simulink model "gm_parallel_phase_voltages_per_switching_state_6_vnl"  (R2022a)
settings: Solver=FixedStepDiscrete  StartTime=0.0  StopTime=10.0  RelTol=1e-3
undefined symbols (not defined in the file or in its folder): f_c, Rt, u_dc
libraries: hdlmdlgenlib x82, simulink x6, hdlsllib x2
(part 1 of 7)
settings Model: Creator=Andre Merx  LastModifiedBy=Andre Merx
settings SolverCC: AlgebraicLoopSolver=TrustRegion
settings DataIOCC: LimitDataPoints=on  SaveOutput=off  SaveTime=off
settings OptimizationCC: BlockReduction=off  ConditionallyExecuteInputs=off  DefaultParameterBehavior=Inlined  LifeSpan=inf
settings DebuggingCC: AlgebraicLoopMsg=error  InheritedTsInSrcMsg=none  SingleTaskRateTransMsg=error  UnconnectedInputMsg=warning  UnconnectedOutputMsg=warning  UnconnectedLineMsg=warning  AllowSymbolicDim=off  StrictBusMsg=ErrorOnBusTreatedAsVector  SFUnexpectedBacktrackingDiag=warning  SFNoUnconditionalDefaultTransitionDiag=warning  SFExecutionAtInitializationDiag=none  SFMachineParentedDataDiag=warning  ArithmeticOperatorsInVariantConditions=warning
settings HardwareCC: ProdBitPerPointer=32  ProdBitPerSizeT=32  ProdBitPerPtrDiffT=32  ProdLargestAtomicFloat=None  ProdIntDivRoundTo=Undefined  ProdEndianess=Unspecified  ProdWordSize=32  ProdHWDeviceType=ASIC/FPGA->ASIC/FPGA  ProdEqTarget=off
settings SFSimCC: SimUseLocalCustomCode=off  CustomCodeUndefinedFunction=UseInterfaceOnly
settings RTWCC: RTWUseLocalCustomCode=off
settings CodeAppCC: StateflowObjectComments=on
settings GRTTargetCC: TargetLangStandard=C89/C90 (ANSI)
settings ConfigComp: CovScope=ReferencedModels  CovMetricSettings=dw  CovSaveCumulativeToWorkspaceVar=on  CovSaveSingleToWorkspaceVar=on  CovExternalEMLEnable=off  CovSFcnEnable=off

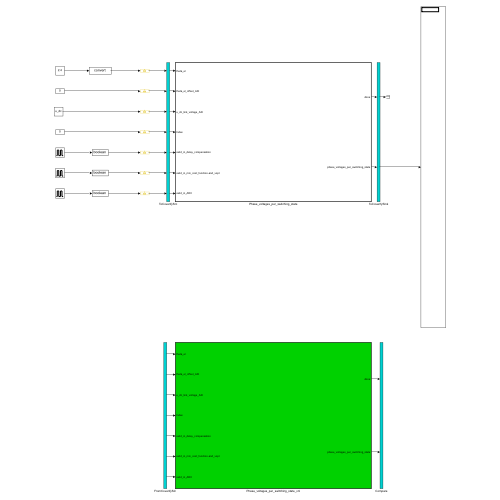
[thumbnail: Simulink's stored preview of the top-level diagram]
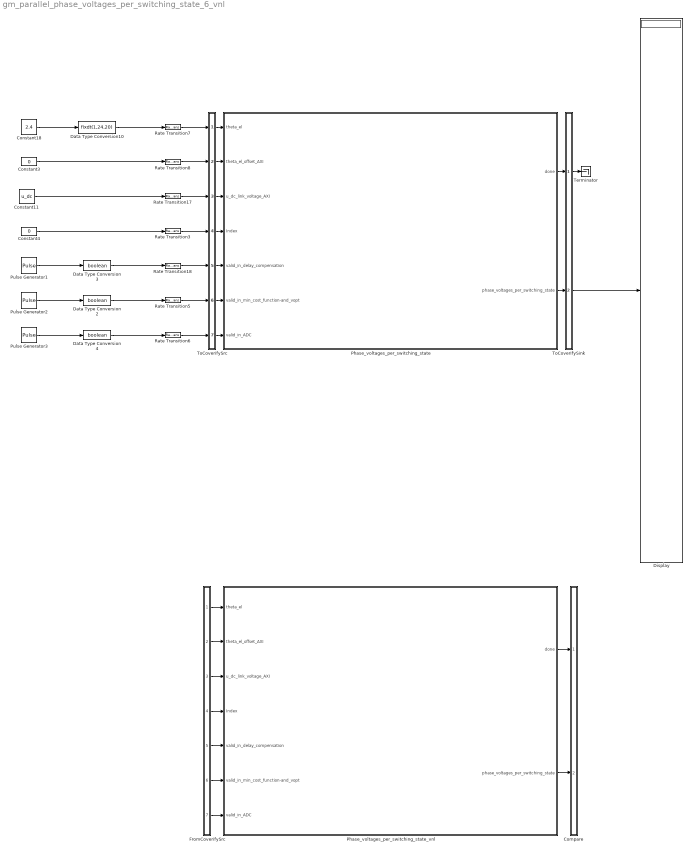
== system gm_parallel_phase_voltages_per_switching_state_6_vnl ==
  Compare : Subsystem
      mask Display: disp('')
  Constant11 : Constant  Value=u_dc  OutDataTypeStr=single  SampleTime=-1
  Constant18 : Constant  Value=2.4
  Constant3 : Constant  Value=0  OutDataTypeStr=single  SampleTime=-1
  Constant4 : Constant  Value=0  OutDataTypeStr=int32  SampleTime=-1
  Data Type Conversion10 : DataTypeConversion  OutDataTypeStr=fixdt(1,24,20)  SaturateOnIntegerOverflow=off  RndMeth=Floor
  Data Type Conversion2 : DataTypeConversion  OutDataTypeStr=boolean  SaturateOnIntegerOverflow=off  RndMeth=Floor
  Data Type Conversion3 : DataTypeConversion  OutDataTypeStr=boolean  SaturateOnIntegerOverflow=off  RndMeth=Floor
  Data Type Conversion4 : DataTypeConversion  OutDataTypeStr=boolean  SaturateOnIntegerOverflow=off  RndMeth=Floor
  Display : Display
  FromCoverifySrc : Subsystem
      mask Display: disp('')
  Phase_voltages_per_switching_state : Subsystem  TreatAsAtomicUnit=on
  Phase_voltages_per_switching_state_vnl : Subsystem  TreatAsAtomicUnit=on
  Pulse Generator1 : DiscretePulseGenerator  PulseType=Time based  Period=1/f_c
  Pulse Generator2 : DiscretePulseGenerator  PulseType=Time based  Period=1/f_c
  Pulse Generator3 : DiscretePulseGenerator  PulseType=Time based  Period=1/f_c
  Rate Transition{3,5..8,17..18} (7 alike) : RateTransition  OutPortSampleTime=Rt
  Terminator : Terminator
  ToCoverifySink : Subsystem
      mask Display: disp('')
  ToCoverifySrc : Subsystem
      mask Display: disp('')
  wires:
  Data Type Conversion2/1 -> Rate Transition5/1
  Data Type Conversion3/1 -> Rate Transition18/1
  Data Type Conversion4/1 -> Rate Transition6/1
  Pulse Generator3/1 -> Data Type Conversion4/1
  Pulse Generator2/1 -> Data Type Conversion2/1
  Constant18/1 -> Data Type Conversion10/1
  Pulse Generator1/1 -> Data Type Conversion3/1
  Constant4/1 -> Rate Transition3/1
  Constant3/1 -> Rate Transition8/1
  Constant11/1 -> Rate Transition17/1
  Data Type Conversion10/1 -> Rate Transition7/1
  ToCoverifySrc/1(out1) -> Phase_voltages_per_switching_state/1(theta_el)
  ToCoverifySrc/2(out2) -> Phase_voltages_per_switching_state/2(theta_el_offset_AXI)
  ToCoverifySrc/3(out3) -> Phase_voltages_per_switching_state/3(u_dc_link_voltage_AXI)
  ToCoverifySrc/4(out4) -> Phase_voltages_per_switching_state/4(Index)
  ToCoverifySrc/5(out5) -> Phase_voltages_per_switching_state/5(valid_in_delay_compensation)
  ToCoverifySrc/6(out6) -> Phase_voltages_per_switching_state/6(valid_in_min_cost_function-and_vopt)
  ToCoverifySrc/7(out7) -> Phase_voltages_per_switching_state/7(valid_in_ADC)
  Phase_voltages_per_switching_state/1(done) -> ToCoverifySink/1(in1)
  Phase_voltages_per_switching_state/2(phase_voltages_per_switching_state) -> ToCoverifySink/2(in2)
  Rate Transition7/1 -> ToCoverifySrc/1(in1)
  Rate Transition8/1 -> ToCoverifySrc/2(in2)
  Rate Transition17/1 -> ToCoverifySrc/3(in3)
  Rate Transition3/1 -> ToCoverifySrc/4(in4)
  Rate Transition18/1 -> ToCoverifySrc/5(in5)
  Rate Transition5/1 -> ToCoverifySrc/6(in6)
  Rate Transition6/1 -> ToCoverifySrc/7(in7)
  ToCoverifySink/1(out1) -> Terminator/1
  ToCoverifySink/2(out2) -> Display/1
  FromCoverifySrc/1(out1) -> Phase_voltages_per_switching_state_vnl/1(theta_el)
  FromCoverifySrc/2(out2) -> Phase_voltages_per_switching_state_vnl/2(theta_el_offset_AXI)
  FromCoverifySrc/3(out3) -> Phase_voltages_per_switching_state_vnl/3(u_dc_link_voltage_AXI)
  FromCoverifySrc/4(out4) -> Phase_voltages_per_switching_state_vnl/4(Index)
  FromCoverifySrc/5(out5) -> Phase_voltages_per_switching_state_vnl/5(valid_in_delay_compensation)
  FromCoverifySrc/6(out6) -> Phase_voltages_per_switching_state_vnl/6(valid_in_min_cost_function-and_vopt)
  FromCoverifySrc/7(out7) -> Phase_voltages_per_switching_state_vnl/7(valid_in_ADC)
  Phase_voltages_per_switching_state_vnl/1(done) -> Compare/1(in1)
  Phase_voltages_per_switching_state_vnl/2(phase_voltages_per_switching_state) -> Compare/2(in2)

== system gm_parallel_phase_voltages_per_switching_state_6_vnl/Compare ==
  in1 : Inport
  in2 : Inport  Port=2
  Assert_done : Subsystem
  Assert_phase_voltages_per_switching_state : Subsystem
  CleanupScopes : Subsystem
      settings: OpenFcn=|
      | blkName = gcb; %self block
      | idx = regexp(blkName, '/CleanupScopes$', 'once');
      | blkParent = blkName(1:idx-1);
      | blks=find_system(blkParent, 'LookUnderMasks', 'all','blocktype', 'Scope');
      | for itr = 1:length(blks)
      | 	 hScopeCfg = get_param(blks{itr},'ScopeConfiguration');
      | 	 hScopeCfg.Visible = ~ hScopeCfg.Visible;
      | end
      | drawnow;
      mask Display: fprintf(message('hdlcoder:cosim:vnl_dblclick').getString());
  Enable : Subsystem
      settings: OpenFcn=|
      | blkName = gcb;
      | idx = regexp(blkName, '/Enable$', 'once');
      | blkParent = blkName(1:idx-1);
      | blks=find_system(blkParent, 'LookUnderMasks', 'all','blocktype', 'Assertion');
      | e = get_param(blks{1}, 'Enabled');
      | if strcmp(e, 'on'), f= 'off';, else, f = 'on';, end
      | for ii=1:length(blks), set_param(blks{ii}, 'Enabled', f);, end
      | set_param(gcb, 'MaskDisplay',['fprintf(message(''hdlcoder:cosim:vnl_dblclick_assertions'',','''',upper(e),'''',').getString())']);
      mask Display: fprintf(message('hdlcoder:cosim:vnl_dblclick_assertions','OFF').getString());
  pathdelay1 : Delay  DelayLength=68
  pathdelay2 : Delay  DelayLength=68
  wires:
  in1/1 -> pathdelay1/1
  pathdelay1/1 -> Assert_done/1(cosim)
  [out1] -> Assert_done/2(dut)
  in2/1 -> pathdelay2/1
  pathdelay2/1 -> Assert_phase_voltages_per_switching_state/1(cosim)
  [out2] -> Assert_phase_voltages_per_switching_state/2(dut)

== system gm_parallel_phase_voltages_per_switching_state_6_vnl/FromCoverifySrc ==
  out1 : Outport
  out2 : Outport  Port=2
  out3 : Outport  Port=3
  out4 : Outport  Port=4
  out5 : Outport  Port=5
  out6 : Outport  Port=6
  out7 : Outport  Port=7
  wires:
  [in1] -> out1/1
  [in2] -> out2/1
  [in3] -> out3/1
  [in4] -> out4/1
  [in5] -> out5/1
  [in6] -> out6/1
  [in7] -> out7/1

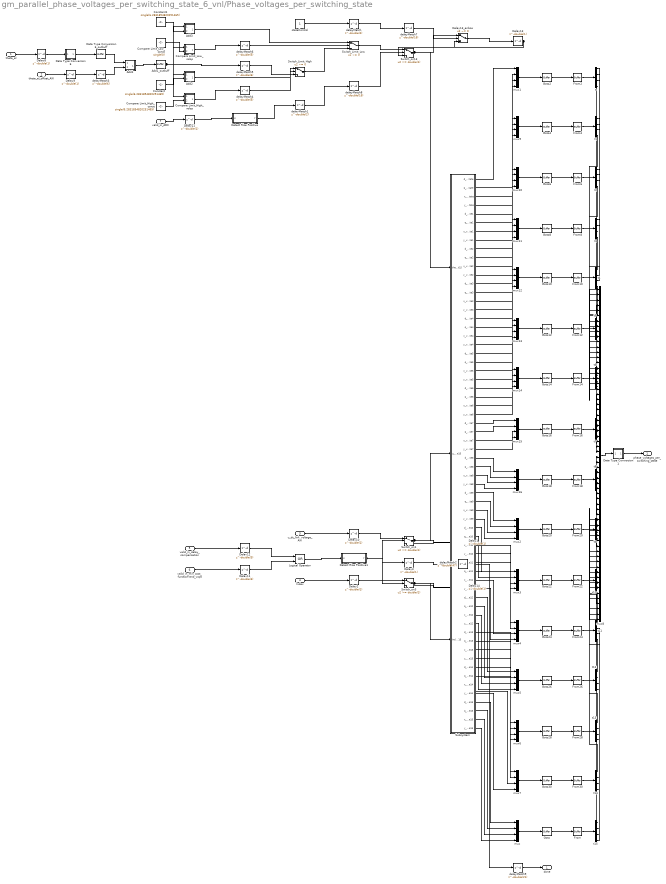
== system gm_parallel_phase_voltages_per_switching_state_6_vnl/Phase_voltages_per_switching_state ==
  theta_el : Inport  OutDataTypeStr=fixdt(1, 24, 20)  PortDimensions=1  SampleTime=1e-08
  theta_el_offset_AXI : Inport  Port=2  OutDataTypeStr=single  PortDimensions=1  SampleTime=1e-08
  u_dc_link_voltage_AXI : Inport  Port=3  OutDataTypeStr=single  PortDimensions=1  SampleTime=1e-08
  Index : Inport  Port=4  OutDataTypeStr=int32  PortDimensions=1  SampleTime=1e-08
  valid_in_delay_compensation : Inport  Port=5  OutDataTypeStr=boolean  PortDimensions=1  SampleTime=1e-08
  valid_in_min_cost_function-and_vopt : Inport  Port=6  OutDataTypeStr=boolean  PortDimensions=1  SampleTime=1e-08
  valid_in_ADC : Inport  Port=7  OutDataTypeStr=boolean  PortDimensions=1  SampleTime=1e-08
  Add1 : Subsystem
      mask Display: disp('NFP\nadd');
  Add1_outbuff : hdlmdlgenlib/Buffer
      settings: SourceProductBaseCode=SL
  Add2 : Subsystem
      mask Display: disp('NFP\nadd');
  Add3 : Subsystem
      mask Display: disp('NFP\nadd');
  Compare Limit_High_const : Constant  Value=single(6.2831854820251465)  OutDataTypeStr=single  SampleTime=1e-08
  Compare Limit_High_relop : Subsystem
      mask Display: disp('NFP\nrelop');
  Compare Limit_Low_const : Constant  Value=single(0)  OutDataTypeStr=single  SampleTime=1e-08
  Compare Limit_Low_relop : Subsystem
      mask Display: disp('NFP\nrelop');
  Constant : Constant  Value=single(6.2831854820251465)  OutDataTypeStr=single  SampleTime=1e-08
  Constant1 : Constant  Value=single(6.2831854820251465)  OutDataTypeStr=single  SampleTime=1e-08
  Data Type Conversion1 : Subsystem
      mask Display: disp('NFP\nconv');
  Data Type Conversion6 : Subsystem
      mask Display: disp('NFP\nconv');
  Data Type Conversion6_outbuff : hdlmdlgenlib/Buffer
      settings: SourceProductBaseCode=SL
  Delay{1..3,8..10,13..14,21} (9 alike) : Delay  DelayLength=double(1)  InitialCondition=0  SampleTime=1e-08
  Delay11 : Delay  DelayLength=double(3)  InitialCondition=0  SampleTime=1e-08
  Delay12 : Delay  DelayLength=double(3)  InitialCondition=0  SampleTime=1e-08
  Delay13_enbsw : Switch  Criteria=u2 ~= 0  Threshold=double(0)  OutDataTypeStr=single  SampleTime=1e-08  SaturateOnIntegerOverflow=off  InputSameDT=off
  Detect Rise Positive : Subsystem  mask(Detect Rise Positive){vinit=double(0), InputProcessing=Elements as channels (sample based), OutDataTypeStr=boolean}
      mask prompts: vinit "Simulink:masks:InitialCondition_MP"; InputProcessing "Simulink:masks:InputProcessing_MP"; OutDataTypeStr "Simulink:masks:OutputDataType_MP"
      mask help: Simulink:masks:DetectRisePositive_MD
      mask init:
      | InputProcessing = 'Elements as channels (sample based)';
      | OutDataTypeStr = 'boolean';
      | vinit = double(0);
      mask TypeOptions InputProcessing: Simulink:masks:ColumnsAsChannelsFrameBased | Simulink:masks:ElementsAsChannelsSampleBased
      mask TypeOptions OutDataTypeStr: Simulink:masks:uint8 | Simulink:masks:boolean
      mask Display: fprintf('U > 0\n&  NOT\nU/z > 0')
  Detect Rise Positive1 : Subsystem  mask(Detect Rise Positive){vinit=double(0), InputProcessing=Elements as channels (sample based), OutDataTypeStr=boolean}
      mask prompts: vinit "Simulink:masks:InitialCondition_MP"; InputProcessing "Simulink:masks:InputProcessing_MP"; OutDataTypeStr "Simulink:masks:OutputDataType_MP"
      mask help: Simulink:masks:DetectRisePositive_MD
      mask init:
      | InputProcessing = 'Elements as channels (sample based)';
      | OutDataTypeStr = 'boolean';
      | vinit = double(0);
      mask TypeOptions InputProcessing: Simulink:masks:ColumnsAsChannelsFrameBased | Simulink:masks:ElementsAsChannelsSampleBased
      mask TypeOptions OutDataTypeStr: Simulink:masks:uint8 | Simulink:masks:boolean
      mask Display: fprintf('U > 0\n&  NOT\nU/z > 0')
  From{,2,4,6,8,10,12,14,16,18,20,22,24,26,28,30} (16 alike) : hdlmdlgenlib/Buffer
      settings: SourceProductBaseCode=SL
  Goto{,2,4,6,8,10,12,14,16,18,20,22,24,26,28,30} (16 alike) : hdlmdlgenlib/Buffer
      settings: SourceProductBaseCode=SL
  Logical Operator : Logic  Operator=OR  AllPortsSameDT=off  OutDataTypeStr=boolean  SampleTime=1e-08
  Subsystem : Subsystem
  Switch_Limit_High : Switch  Criteria=u2 ~= 0  Threshold=double(0)  OutDataTypeStr=single  SampleTime=1e-08  SaturateOnIntegerOverflow=off  InputSameDT=off
  Switch_Limit_Low : Switch  Criteria=u2 ~= 0  Threshold=double(0)  OutDataTypeStr=single  SampleTime=1e-08  SaturateOnIntegerOverflow=off  InputSameDT=off
  Switch_on1 : Switch  Threshold=double(1)  OutDataTypeStr=single  RndMeth=Simplest  SampleTime=1e-08  SaturateOnIntegerOverflow=off  InputSameDT=off
  Switch_on13 : Switch  Threshold=double(1)  OutDataTypeStr=single  RndMeth=Simplest  SampleTime=1e-08  SaturateOnIntegerOverflow=off  InputSameDT=off
  Switch_on3 : Switch  Threshold=double(1)  OutDataTypeStr=int32  RndMeth=Simplest  SampleTime=1e-08  SaturateOnIntegerOverflow=off  InputSameDT=off
  delayMatch : Delay  DelayLength=double(2)  InitialCondition=0  SampleTime=1e-08
  delayMatch1 : Delay  DelayLength=double(2)  InitialCondition=0  SampleTime=1e-08
  delayMatch2 : Delay  DelayLength=double(47)  InitialCondition=0  SampleTime=1e-08
  delayMatch3 : Delay  DelayLength=double(6)  InitialCondition=0  SampleTime=1e-08
  delayMatch4 : Delay  DelayLength=double(5)  InitialCondition=0  SampleTime=1e-08
  delayMatch5 : Delay  DelayLength=double(6)  InitialCondition=0  SampleTime=1e-08
  delayMatch6 : Delay  DelayLength=double(5)  InitialCondition=0  SampleTime=1e-08
  delayMatch7 : Delay  DelayLength=double(16)  InitialCondition=0  SampleTime=1e-08
  delayMatch8 : Delay  DelayLength=double(16)  InitialCondition=0  SampleTime=1e-08
  delayMatch9 : Delay  DelayLength=double(21)  InitialCondition=0  SampleTime=1e-08
  mux{,1..7,9..16} (16 alike) : Mux
  mux8 : Mux  Inputs=64
  stateControl : Constant  OutDataTypeStr=boolean  SampleTime=1e-08
  t{,1..15} (16 alike) : Demux
  done : Outport  SampleTime=1e-08
  phase_voltages_per_switching_state : Outport  Port=2  SampleTime=1e-08
  wires:
  Delay14/1 -> Switch_on3/3
  Delay1/1 -> Switch_on1/3
  Delay13/1 -> Delay13_enbsw/3, Switch_on13/3
  Delay13_enbsw/1 -> Delay13/1
  Switch_on13/1 -> Delay13_enbsw/1, Subsystem/1(theta_el_with_offset15)
  delayMatch2/1 -> delayMatch9/1
  delayMatch1/1 -> delayMatch8/1
  delayMatch/1 -> delayMatch7/1
  Delay9/1 -> delayMatch3/1
  Data Type Conversion6/1(Out1) -> Data Type Conversion6_outbuff/1
  Data Type Conversion1/1(Out1) -> phase_voltages_per_switching_state/1
  Compare Limit_Low_relop/1(Out1) -> delayMatch6/1
  Compare Limit_High_relop/1(Out1) -> delayMatch4/1
  Add3/1(Out1) -> Switch_Limit_Low/1
  Add2/1(Out1) -> Switch_Limit_High/1
  Add1/1(Out1) -> Add1_outbuff/1
  Delay3/1 -> delayMatch2/1
  Detect Rise Positive/1(Y) -> delayMatch1/1
  stateControl/1 -> delayMatch/1
  delayMatch7/1 -> Delay13_enbsw/2
  t15/4 -> mux8/64
  t15/3 -> mux8/63
  t15/2 -> mux8/62
  t15/1 -> mux8/61
  t14/4 -> mux8/60
  t14/3 -> mux8/59
  t14/2 -> mux8/58
  t14/1 -> mux8/57
  t13/4 -> mux8/56
  t13/3 -> mux8/55
  t13/2 -> mux8/54
  t13/1 -> mux8/53
  t12/4 -> mux8/52
  t12/3 -> mux8/51
  t12/2 -> mux8/50
  t12/1 -> mux8/49
  t11/4 -> mux8/48
  t11/3 -> mux8/47
  t11/2 -> mux8/46
  t11/1 -> mux8/45
  t10/4 -> mux8/44
  t10/3 -> mux8/43
  t10/2 -> mux8/42
  t10/1 -> mux8/41
  t9/4 -> mux8/40
  t9/3 -> mux8/39
  t9/2 -> mux8/38
  t9/1 -> mux8/37
  t8/4 -> mux8/36
  t8/3 -> mux8/35
  t8/2 -> mux8/34
  t8/1 -> mux8/33
  t7/4 -> mux8/32
  t7/3 -> mux8/31
  t7/2 -> mux8/30
  t7/1 -> mux8/29
  t6/4 -> mux8/28
  t6/3 -> mux8/27
  t6/2 -> mux8/26
  t6/1 -> mux8/25
  t5/4 -> mux8/24
  t5/3 -> mux8/23
  t5/2 -> mux8/22
  t5/1 -> mux8/21
  t4/4 -> mux8/20
  t4/3 -> mux8/19
  t4/2 -> mux8/18
  t4/1 -> mux8/17
  t3/4 -> mux8/16
  t3/3 -> mux8/15
  t3/2 -> mux8/14
  t3/1 -> mux8/13
  t2/4 -> mux8/12
  t2/3 -> mux8/11
  t2/2 -> mux8/10
  t2/1 -> mux8/9
  t1/4 -> mux8/8
  t1/3 -> mux8/7
  t1/2 -> mux8/6
  t1/1 -> mux8/5
  t/4 -> mux8/4
  t/3 -> mux8/3
  t/2 -> mux8/2
  t/1 -> mux8/1
  Compare Limit_Low_const/1 -> Compare Limit_Low_relop/2(In2)
  Compare Limit_High_const/1 -> Compare Limit_High_relop/2(In2)
  delayMatch6/1 -> Switch_Limit_Low/2
  delayMatch4/1 -> Switch_Limit_High/2
  Add1_outbuff/1 -> delayMatch5/1, Add2/1(In1), Add3/1(In1), Compare Limit_High_relop/1(In1), Compare Limit_Low_relop/1(In1)
  Goto8/1 -> From8/1
  Goto6/1 -> From6/1
  Goto4/1 -> From4/1
  Goto30/1 -> From30/1
  Goto28/1 -> From28/1
  Goto26/1 -> From26/1
  Goto24/1 -> From24/1
  Goto22/1 -> From22/1
  Goto20/1 -> From20/1
  Goto2/1 -> From2/1
  Goto18/1 -> From18/1
  Goto16/1 -> From16/1
  Goto14/1 -> From14/1
  Goto12/1 -> From12/1
  Goto10/1 -> From10/1
  Goto/1 -> From/1
  Switch_on3/1 -> Delay14/1, Subsystem/3(Index 15)
  Switch_on1/1 -> Delay1/1, Subsystem/2(u_dc_link_voltage15)
  Switch_Limit_Low/1 -> Switch_on13/1
  Switch_Limit_High/1 -> Switch_Limit_Low/3
  Subsystem/64(y_voltage_per_switching_state15) -> mux/4
  Subsystem/63(x_voltage_per_switching_state15) -> mux/3
  Subsystem/62(q_voltage_per_switching_state15) -> mux/2
  Subsystem/61(d_voltage_per_switching_state15) -> mux/1
  Subsystem/60(y_voltage_per_switching_state14) -> mux7/4
  Subsystem/59(x_voltage_per_switching_state14) -> mux7/3
  Subsystem/58(q_voltage_per_switching_state14) -> mux7/2
  Subsystem/57(d_voltage_per_switching_state14) -> mux7/1
  Subsystem/56(y_voltage_per_switching_state13) -> mux6/4
  Subsystem/55(x_voltage_per_switching_state13) -> mux6/3
  Subsystem/54(q_voltage_per_switching_state13) -> mux6/2
  Subsystem/53(d_voltage_per_switching_state13) -> mux6/1
  Subsystem/52(y_voltage_per_switching_state12) -> mux5/4
  Subsystem/51(x_voltage_per_switching_state12) -> mux5/3
  Subsystem/50(q_voltage_per_switching_state12) -> mux5/2
  Subsystem/49(d_voltage_per_switching_state12) -> mux5/1
  Subsystem/48(y_voltage_per_switching_state11) -> mux4/4
  Subsystem/47(x_voltage_per_switching_state11) -> mux4/3
  Subsystem/46(q_voltage_per_switching_state11) -> mux4/2
  Subsystem/45(d_voltage_per_switching_state11) -> mux4/1
  Subsystem/44(y_voltage_per_switching_state10) -> mux3/4
  Subsystem/43(x_voltage_per_switching_state10) -> mux3/3
  Subsystem/42(q_voltage_per_switching_state10) -> mux3/2
  Subsystem/41(d_voltage_per_switching_state10) -> mux3/1
  Subsystem/40(y_voltage_per_switching_state9) -> mux2/4
  Subsystem/39(x_voltage_per_switching_state9) -> mux2/3
  Subsystem/38(q_voltage_per_switching_state9) -> mux2/2
  Subsystem/37(d_voltage_per_switching_state9) -> mux2/1
  Subsystem/36(y_voltage_per_switching_state8) -> mux16/4
  Subsystem/35(x_voltage_per_switching_state8) -> mux16/3
  Subsystem/34(q_voltage_per_switching_state8) -> mux16/2
  Subsystem/33(d_voltage_per_switching_state8) -> mux16/1
  Subsystem/32(y_voltage_per_switching_state7) -> mux15/4
  Subsystem/31(x_voltage_per_switching_state7) -> mux15/3
  Subsystem/30(q_voltage_per_switching_state7) -> mux15/2
  Subsystem/29(d_voltage_per_switching_state7) -> mux15/1
  Subsystem/28(y_voltage_per_switching_state6) -> mux14/4
  Subsystem/27(x_voltage_per_switching_state6) -> mux14/3
  Subsystem/26(q_voltage_per_switching_state6) -> mux14/2
  Subsystem/25(d_voltage_per_switching_state6) -> mux14/1
  Subsystem/24(y_voltage_per_switching_state5) -> mux13/4
  Subsystem/23(x_voltage_per_switching_state5) -> mux13/3
  Subsystem/22(q_voltage_per_switching_state5) -> mux13/2
  Subsystem/21(d_voltage_per_switching_state5) -> mux13/1
  Subsystem/20(y_voltage_per_switching_state4) -> mux12/4
  Subsystem/19(x_voltage_per_switching_state4) -> mux12/3
  Subsystem/18(q_voltage_per_switching_state4) -> mux12/2
  Subsystem/17(d_voltage_per_switching_state4) -> mux12/1
  Subsystem/16(y_voltage_per_switching_state3) -> mux11/4
  Subsystem/15(x_voltage_per_switching_state3) -> mux11/3
  Subsystem/14(q_voltage_per_switching_state3) -> mux11/2
  Subsystem/13(d_voltage_per_switching_state3) -> mux11/1
  Subsystem/12(y_voltage_per_switching_state2) -> mux10/4
  Subsystem/11(x_voltage_per_switching_state2) -> mux10/3
  Subsystem/10(q_voltage_per_switching_state2) -> mux10/2
  Subsystem/9(d_voltage_per_switching_state2) -> mux10/1
  Subsystem/8(y_voltage_per_switching_state1) -> mux9/4
  Subsystem/7(x_voltage_per_switching_state1) -> mux9/3
  Subsystem/6(q_voltage_per_switching_state1) -> mux9/2
  Subsystem/5(d_voltage_per_switching_state1) -> mux9/1
  Subsystem/4(y_voltage_per_switching_state) -> mux1/4
  Subsystem/3(x_voltage_per_switching_state) -> mux1/3
  Subsystem/2(q_voltage_per_switching_state) -> mux1/2
  Subsystem/1(d_voltage_per_switching_state) -> mux1/1
  mux16/1 -> Goto18/1
  mux15/1 -> Goto16/1
  mux14/1 -> Goto14/1
  mux13/1 -> Goto12/1
  mux12/1 -> Goto10/1
  mux11/1 -> Goto8/1
  mux10/1 -> Goto6/1
  mux9/1 -> Goto4/1
  mux8/1 -> Data Type Conversion1/1(In1)
  mux7/1 -> Goto30/1
  mux6/1 -> Goto28/1
  mux5/1 -> Goto26/1
  mux4/1 -> Goto24/1
  mux3/1 -> Goto22/1
  mux2/1 -> Goto20/1
  mux1/1 -> Goto2/1
  mux/1 -> Goto/1
  Logical Operator/1 -> Detect Rise Positive1/1(U)
  From8/1 -> t3/1
  From6/1 -> t2/1
  From4/1 -> t1/1
  From30/1 -> t14/1
  From28/1 -> t13/1
  From26/1 -> t12/1
  From24/1 -> t11/1
  From22/1 -> t10/1
  From20/1 -> t9/1
  From2/1 -> t/1
  From18/1 -> t8/1
  From16/1 -> t7/1
  From14/1 -> t6/1
  From12/1 -> t5/1
  From10/1 -> t4/1
  From/1 -> t15/1
  Detect Rise Positive1/1(Y) -> Switch_on3/2, Switch_on1/2, Delay3/1
  delayMatch8/1 -> Switch_on13/2
  delayMatch3/1 -> Add1/2(In2)
  Delay8/1 -> Data Type Conversion6/1(In1)
  delayMatch9/1 -> done/1
  Delay21/1 -> Detect Rise Positive/1(U)
  Delay2/1 -> Switch_on3/1
  Delay12/1 -> Logical Operator/1
  Delay11/1 -> Logical Operator/2
  Delay10/1 -> Switch_on1/1
  Data Type Conversion6_outbuff/1 -> Add1/1(In1)
  Constant1/1 -> Add3/2(In2)
  Constant/1 -> Add2/2(In2)
  delayMatch5/1 -> Switch_Limit_High/3
  valid_in_ADC/1 -> Delay21/1
  valid_in_min_cost_function-and_vopt/1 -> Delay11/1
  valid_in_delay_compensation/1 -> Delay12/1
  Index/1 -> Delay2/1
  u_dc_link_voltage_AXI/1 -> Delay10/1
  theta_el_offset_AXI/1 -> Delay9/1
  theta_el/1 -> Delay8/1

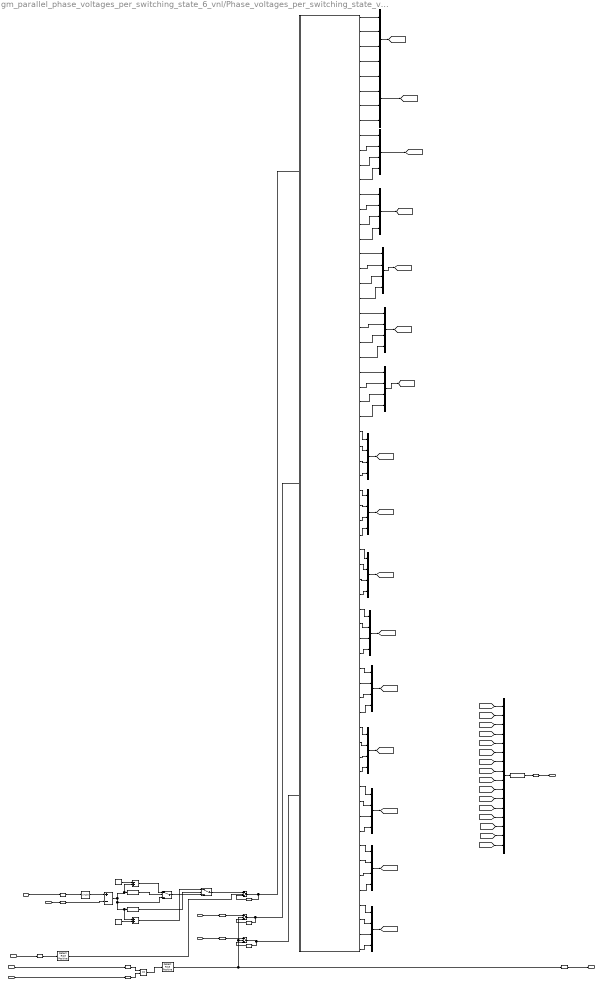
== system gm_parallel_phase_voltages_per_switching_state_6_vnl/Phase_voltages_per_switching_state_vnl ==
  theta_el : Inport
  theta_el_offset_AXI : Inport  Port=2
  u_dc_link_voltage_AXI : Inport  Port=3
  Index : Inport  Port=4
  valid_in_delay_compensation : Inport  Port=5
  valid_in_min_cost_function-and_vopt : Inport  Port=6
  valid_in_ADC : Inport  Port=7
  Add1 : Sum  Inputs=+-  OutDataTypeStr=Inherit: Same as accumulator
  Add2 : Sum  Inputs=-+  OutDataTypeStr=Inherit: Same as first input
  Add3 : Sum  OutDataTypeStr=Inherit: Same as first input
  Compare Limit_High : simulink/Logic and Bit Operations/Compare To Constant  relop=>=  const=2*pi  OutDataTypeStr=boolean
  Compare Limit_Low : simulink/Logic and Bit Operations/Compare To Constant  relop=<  const=0  OutDataTypeStr=boolean
  Constant : Constant  Value=2*pi  OutDataTypeStr=single  SampleTime=Rt
  Constant1 : Constant  Value=2*pi  OutDataTypeStr=single  SampleTime=Rt
  Data Type Conversion1 : DataTypeConversion  OutDataTypeStr=fixdt(1,24,11)  SaturateOnIntegerOverflow=off  RndMeth=Floor
  Data Type Conversion6 : DataTypeConversion  OutDataTypeStr=single  RndMeth=Nearest  SaturateOnIntegerOverflow=off
  Delay{1..4,8..10,13..14,21} (10 alike) : Delay  DelayLength=1
  Delay11 : Delay  DelayLength=3
  Delay12 : Delay  DelayLength=3
  Detect Rise Positive : hdlsllib/Logic and Bit Operations/Detect Rise Positive  vinit=0  OutDataTypeStr=boolean
      settings: SourceProductBaseCode=SL
  Detect Rise Positive1 : hdlsllib/Logic and Bit Operations/Detect Rise Positive  vinit=0  OutDataTypeStr=boolean
      settings: SourceProductBaseCode=SL
  Logical Operator : Logic  Operator=OR  AllPortsSameDT=off  OutDataTypeStr=boolean
  Mux{,1..15} (16 alike) : Mux
  Mux16 : Mux  Inputs=16
  Subsystem : Subsystem
  Switch_Limit_High : Switch  Criteria=u2 > Threshold  OutDataTypeStr=single  SaturateOnIntegerOverflow=off  InputSameDT=off
  Switch_Limit_Low : Switch  Criteria=u2 > Threshold  OutDataTypeStr=single  SaturateOnIntegerOverflow=off  InputSameDT=off
  Switch_on1 : Switch  Threshold=1  OutDataTypeStr=single  RndMeth=Simplest  SaturateOnIntegerOverflow=off  InputSameDT=off
  Switch_on13 : Switch  Threshold=1  OutDataTypeStr=single  RndMeth=Simplest  SaturateOnIntegerOverflow=off  InputSameDT=off
  Switch_on3 : Switch  Threshold=1  OutDataTypeStr=Inherit: Inherit via back propagation  RndMeth=Simplest  SaturateOnIntegerOverflow=off  InputSameDT=off
  done : Outport
  phase_voltages_per_switching_state : Outport  Port=2
  wires:
  Delay4/1 -> phase_voltages_per_switching_state/1
  [voltage_16] -> Mux16/16
  [voltage_13] -> Mux16/13
  [voltage_11] -> Mux16/11
  [voltage_9] -> Mux16/9
  [voltage_8] -> Mux16/8
  [voltage_7] -> Mux16/7
  [voltage_6] -> Mux16/6
  [voltage_5] -> Mux16/5
  [voltage_4] -> Mux16/4
  [voltage_3] -> Mux16/3
  [voltage_2] -> Mux16/2
  [voltage_1] -> Mux16/1
  Mux16/1 -> Data Type Conversion1/1
  Data Type Conversion1/1 -> Delay4/1
  [voltage_15] -> Mux16/15
  Mux15/1 -> [voltage_15]
  Subsystem/58(q_voltage_per_switching_state14) -> Mux15/2
  Subsystem/59(x_voltage_per_switching_state14) -> Mux15/3
  Subsystem/60(y_voltage_per_switching_state14) -> Mux15/4
  Subsystem/57(d_voltage_per_switching_state14) -> Mux15/1
  Mux14/1 -> [voltage_14]
  Subsystem/54(q_voltage_per_switching_state13) -> Mux14/2
  Subsystem/55(x_voltage_per_switching_state13) -> Mux14/3
  Subsystem/53(d_voltage_per_switching_state13) -> Mux14/1
  Subsystem/56(y_voltage_per_switching_state13) -> Mux14/4
  [voltage_14] -> Mux16/14
  Subsystem/49(d_voltage_per_switching_state12) -> Mux13/1
  Subsystem/51(x_voltage_per_switching_state12) -> Mux13/3
  Subsystem/50(q_voltage_per_switching_state12) -> Mux13/2
  Subsystem/52(y_voltage_per_switching_state12) -> Mux13/4
  Mux13/1 -> [voltage_13]
  Mux12/1 -> [voltage_12]
  Subsystem/45(d_voltage_per_switching_state11) -> Mux12/1
  Subsystem/47(x_voltage_per_switching_state11) -> Mux12/3
  Subsystem/46(q_voltage_per_switching_state11) -> Mux12/2
  Subsystem/48(y_voltage_per_switching_state11) -> Mux12/4
  [voltage_12] -> Mux16/12
  Subsystem/44(y_voltage_per_switching_state10) -> Mux11/4
  Subsystem/42(q_voltage_per_switching_state10) -> Mux11/2
  Subsystem/41(d_voltage_per_switching_state10) -> Mux11/1
  Subsystem/43(x_voltage_per_switching_state10) -> Mux11/3
  Mux11/1 -> [voltage_11]
  Subsystem/38(q_voltage_per_switching_state9) -> Mux10/2
  Subsystem/37(d_voltage_per_switching_state9) -> Mux10/1
  Subsystem/39(x_voltage_per_switching_state9) -> Mux10/3
  Subsystem/40(y_voltage_per_switching_state9) -> Mux10/4
  Mux10/1 -> [voltage_10]
  [voltage_10] -> Mux16/10
  Subsystem/35(x_voltage_per_switching_state8) -> Mux9/3
  Mux9/1 -> [voltage_9]
  Subsystem/34(q_voltage_per_switching_state8) -> Mux9/2
  Subsystem/33(d_voltage_per_switching_state8) -> Mux9/1
  Subsystem/36(y_voltage_per_switching_state8) -> Mux9/4
  Subsystem/31(x_voltage_per_switching_state7) -> Mux8/3
  Subsystem/30(q_voltage_per_switching_state7) -> Mux8/2
  Subsystem/32(y_voltage_per_switching_state7) -> Mux8/4
  Subsystem/29(d_voltage_per_switching_state7) -> Mux8/1
  Mux8/1 -> [voltage_8]
  Subsystem/26(q_voltage_per_switching_state6) -> Mux7/2
  Subsystem/27(x_voltage_per_switching_state6) -> Mux7/3
  Subsystem/28(y_voltage_per_switching_state6) -> Mux7/4
  Mux7/1 -> [voltage_7]
  Subsystem/25(d_voltage_per_switching_state6) -> Mux7/1
  Mux6/1 -> [voltage_6]
  Subsystem/24(y_voltage_per_switching_state5) -> Mux6/4
  Subsystem/22(q_voltage_per_switching_state5) -> Mux6/2
  Subsystem/21(d_voltage_per_switching_state5) -> Mux6/1
  Subsystem/23(x_voltage_per_switching_state5) -> Mux6/3
  Subsystem/20(y_voltage_per_switching_state4) -> Mux5/4
  Subsystem/17(d_voltage_per_switching_state4) -> Mux5/1
  Subsystem/18(q_voltage_per_switching_state4) -> Mux5/2
  Subsystem/19(x_voltage_per_switching_state4) -> Mux5/3
  Mux5/1 -> [voltage_5]
  Subsystem/14(q_voltage_per_switching_state3) -> Mux4/2
  Subsystem/16(y_voltage_per_switching_state3) -> Mux4/4
  Subsystem/15(x_voltage_per_switching_state3) -> Mux4/3
  Mux4/1 -> [voltage_4]
  Subsystem/13(d_voltage_per_switching_state3) -> Mux4/1
  Subsystem/11(x_voltage_per_switching_state2) -> Mux3/3
  Subsystem/10(q_voltage_per_switching_state2) -> Mux3/2
  Subsystem/9(d_voltage_per_switching_state2) -> Mux3/1
  Subsystem/12(y_voltage_per_switching_state2) -> Mux3/4
  Mux3/1 -> [voltage_3]
  Subsystem/8(y_voltage_per_switching_state1) -> Mux2/4
  Subsystem/6(q_voltage_per_switching_state1) -> Mux2/2
  Subsystem/5(d_voltage_per_switching_state1) -> Mux2/1
  Subsystem/7(x_voltage_per_switching_state1) -> Mux2/3
  Mux2/1 -> [voltage_2]
  Subsystem/3(x_voltage_per_switching_state) -> Mux1/3
  Subsystem/4(y_voltage_per_switching_state) -> Mux1/4
  Subsystem/2(q_voltage_per_switching_state) -> Mux1/2
  Subsystem/1(d_voltage_per_switching_state) -> Mux1/1
  Mux1/1 -> [voltage_1]
  Mux/1 -> [voltage_16]
  Subsystem/64(y_voltage_per_switching_state15) -> Mux/4
  Subsystem/63(x_voltage_per_switching_state15) -> Mux/3
  Subsystem/62(q_voltage_per_switching_state15) -> Mux/2
  Subsystem/61(d_voltage_per_switching_state15) -> Mux/1
  Delay21/1 -> Detect Rise Positive/1
  Detect Rise Positive/1 -> Switch_on13/2  "End_Cycle"
  valid_in_ADC/1 -> Delay21/1
  Switch_on3/1 -> Subsystem/3(Index 15), Delay14/1
  Delay11/1 -> Logical Operator/2
  Logical Operator/1 -> Detect Rise Positive1/1
  valid_in_min_cost_function-and_vopt/1 -> Delay11/1
  Index/1 -> Delay2/1  "End_Cycle"
  Delay2/1 -> Switch_on3/1
  theta_el/1 -> Delay8/1
  Add2/1 -> Switch_Limit_High/1
  Delay3/1 -> done/1
  Constant1/1 -> Add3/2
  Delay1/1 -> Switch_on1/3
  Compare Limit_Low/1 -> Switch_Limit_Low/2
  Detect Rise Positive1/1 -> Delay3/1, Switch_on1/2, Switch_on3/2  "End_Cycle"
  Switch_on1/1 -> Delay1/1, Subsystem/2(u_dc_link_voltage15)
  valid_in_delay_compensation/1 -> Delay12/1
  Add1/1 -> Compare Limit_High/1, Add2/2, Compare Limit_Low/1, Add3/1, Switch_Limit_High/3
  Switch_Limit_Low/1 -> Switch_on13/1  "End_Cycle"
  Data Type Conversion6/1 -> Add1/1  "End_Cycle"
  Add3/1 -> Switch_Limit_Low/1
  Delay9/1 -> Add1/2
  Delay12/1 -> Logical Operator/1
  Delay10/1 -> Switch_on1/1
  Constant/1 -> Add2/1
  Switch_Limit_High/1 -> Switch_Limit_Low/3
  theta_el_offset_AXI/1 -> Delay9/1
  u_dc_link_voltage_AXI/1 -> Delay10/1  "End_Cycle"
  Switch_on13/1 -> Delay13/1, Subsystem/1(theta_el_with_offset15)
  Delay13/1 -> Switch_on13/3
  Delay14/1 -> Switch_on3/3
  Compare Limit_High/1 -> Switch_Limit_High/2
  Delay8/1 -> Data Type Conversion6/1

== system gm_parallel_phase_voltages_per_switching_state_6_vnl/ToCoverifySink ==
  in1 : Inport
  in2 : Inport  Port=2
  out1 : Outport
  out2 : Outport  Port=2
  tag scope: out1=global, out2=global
  wires:
  in1/1 -> out1/1, [out1]
  in2/1 -> out2/1, [out2]

== system gm_parallel_phase_voltages_per_switching_state_6_vnl/ToCoverifySrc ==
  in1 : Inport
  in2 : Inport  Port=2
  in3 : Inport  Port=3
  in4 : Inport  Port=4
  in5 : Inport  Port=5
  in6 : Inport  Port=6
  in7 : Inport  Port=7
  out1 : Outport
  out2 : Outport  Port=2
  out3 : Outport  Port=3
  out4 : Outport  Port=4
  out5 : Outport  Port=5
  out6 : Outport  Port=6
  out7 : Outport  Port=7
  tag scope: in1=global, in2=global, in3=global, in4=global, in5=global, in6=global, in7=global
  wires:
  in1/1 -> out1/1, [in1]
  in2/1 -> out2/1, [in2]
  in3/1 -> out3/1, [in3]
  in4/1 -> out4/1, [in4]
  in5/1 -> out5/1, [in5]
  in6/1 -> out6/1, [in6]
  in7/1 -> out7/1, [in7]

== system gm_parallel_phase_voltages_per_switching_state_6_vnl/Compare/Assert_done ==
  cosim : Inport
  dut : Inport  Port=2
  AssertEq : Assertion  StopWhenAssertionFail=off
  Compare To Zero : simulink/Logic and Bit Operations/Compare To Zero  relop===  OutDataTypeStr=boolean
  Constant1 : Constant  Value=0  OutDataTypeStr=Inherit: Inherit via back propagation  SampleTime=-1
  Counter : simulink/Sources/Counter Free-Running  NumBits=32  tsamp=-1
  IgnoreCycles : Constant  Value=68  OutDataTypeStr=Inherit: Inherit via back propagation  SampleTime=-1
  Relational Operator : RelationalOperator  Operator=<  OutDataTypeStr=boolean  InputSameDT=off
  Relational Operator1 : RelationalOperator  Operator===  OutDataTypeStr=boolean  InputSameDT=off
  Switch : Switch  Criteria=u2 ~= 0  SaturateOnIntegerOverflow=off  InputSameDT=off
  Switch1 : Switch  Criteria=u2 ~= 0  SaturateOnIntegerOverflow=off  InputSameDT=off
  compare: done : Scope  NumInputPorts=3
  wires:
  Compare To Zero/1 -> compare: done/3
  Relational Operator1/1 -> Compare To Zero/1, AssertEq/1  "err"
  Switch1/1 -> compare: done/1, Relational Operator1/1
  Switch/1 -> compare: done/2, Relational Operator1/2
  Constant1/1 -> Switch/1, Switch1/1
  Relational Operator/1 -> Switch/2, Switch1/2
  cosim/1 -> Switch1/3  "cosim"
  dut/1 -> Switch/3  "dut ref"
  Counter/1 -> Relational Operator/1
  IgnoreCycles/1 -> Relational Operator/2

== system gm_parallel_phase_voltages_per_switching_state_6_vnl/Compare/Assert_phase_voltages_per_switching_state ==
  cosim : Inport
  dut : Inport  Port=2
  AssertEq : Assertion  StopWhenAssertionFail=off
  Compare To Zero : simulink/Logic and Bit Operations/Compare To Zero  relop===  OutDataTypeStr=boolean
  Constant1 : Constant  Value=0  OutDataTypeStr=Inherit: Inherit via back propagation  SampleTime=-1
  Counter : simulink/Sources/Counter Free-Running  NumBits=32  tsamp=-1
  IgnoreCycles : Constant  Value=68  OutDataTypeStr=Inherit: Inherit via back propagation  SampleTime=-1
  Relational Operator : RelationalOperator  Operator=<  OutDataTypeStr=boolean  InputSameDT=off
  Relational Operator1 : RelationalOperator  Operator===  OutDataTypeStr=boolean  InputSameDT=off
  Switch : Switch  Criteria=u2 ~= 0  SaturateOnIntegerOverflow=off  InputSameDT=off
  Switch1 : Switch  Criteria=u2 ~= 0  SaturateOnIntegerOverflow=off  InputSameDT=off
  compare: phase_voltages_per_switching_state : Scope  NumInputPorts=3
  wires:
  Compare To Zero/1 -> compare: phase_voltages_per_switching_state/3
  Relational Operator1/1 -> Compare To Zero/1, AssertEq/1  "err"
  Switch1/1 -> compare: phase_voltages_per_switching_state/1, Relational Operator1/1
  Switch/1 -> compare: phase_voltages_per_switching_state/2, Relational Operator1/2
  Constant1/1 -> Switch/1, Switch1/1
  Relational Operator/1 -> Switch/2, Switch1/2
  cosim/1 -> Switch1/3  "cosim"
  dut/1 -> Switch/3  "dut ref"
  Counter/1 -> Relational Operator/1
  IgnoreCycles/1 -> Relational Operator/2

== system gm_parallel_phase_voltages_per_switching_state_6_vnl/Compare/CleanupScopes ==

== system gm_parallel_phase_voltages_per_switching_state_6_vnl/Compare/Enable ==

== system gm_parallel_phase_voltages_per_switching_state_6_vnl/Phase_voltages_per_switching_state/Add1 ==
  In1 : Inport
  In2 : Inport  Port=2
  Add1 : Sum  Inputs=+-  OutDataTypeStr=single  SampleTime=1e-08
  Add1_pd1 : Delay  DelayLength=6
  Out1 : Outport
  wires:
  Add1_pd1/1 -> Out1/1
  Add1/1 -> Add1_pd1/1
  In2/1 -> Add1/2
  In1/1 -> Add1/1

== system gm_parallel_phase_voltages_per_switching_state_6_vnl/Phase_voltages_per_switching_state/Add2 ==
  In1 : Inport
  In2 : Inport  Port=2
  Add2 : Sum  Inputs=+-  OutDataTypeStr=single  SampleTime=1e-08
  Add2_pd1 : Delay  DelayLength=6
  Out1 : Outport
  wires:
  Add2_pd1/1 -> Out1/1
  Add2/1 -> Add2_pd1/1
  In2/1 -> Add2/2
  In1/1 -> Add2/1

== system gm_parallel_phase_voltages_per_switching_state_6_vnl/Phase_voltages_per_switching_state/Add3 ==
  In1 : Inport
  In2 : Inport  Port=2
  Add3 : Sum  OutDataTypeStr=single  SampleTime=1e-08
  Add3_pd1 : Delay  DelayLength=6
  Out1 : Outport
  wires:
  Add3_pd1/1 -> Out1/1
  Add3/1 -> Add3_pd1/1
  In2/1 -> Add3/2
  In1/1 -> Add3/1

== system gm_parallel_phase_voltages_per_switching_state_6_vnl/Phase_voltages_per_switching_state/Compare Limit_High_relop ==
  In1 : Inport
  In2 : Inport  Port=2
  Compare Limit_High_relop : RelationalOperator  OutDataTypeStr=boolean  SampleTime=1e-08
  Compare Limit_High_relop_pd1 : Delay  DelayLength=1
  Out1 : Outport
  wires:
  Compare Limit_High_relop_pd1/1 -> Out1/1
  Compare Limit_High_relop/1 -> Compare Limit_High_relop_pd1/1
  In2/1 -> Compare Limit_High_relop/2
  In1/1 -> Compare Limit_High_relop/1

== system gm_parallel_phase_voltages_per_switching_state_6_vnl/Phase_voltages_per_switching_state/Compare Limit_Low_relop ==
  In1 : Inport
  In2 : Inport  Port=2
  Compare Limit_Low_relop : RelationalOperator  Operator=<  OutDataTypeStr=boolean  SampleTime=1e-08
  Compare Limit_Low_relop_pd1 : Delay  DelayLength=1
  Out1 : Outport
  wires:
  Compare Limit_Low_relop_pd1/1 -> Out1/1
  Compare Limit_Low_relop/1 -> Compare Limit_Low_relop_pd1/1
  In2/1 -> Compare Limit_Low_relop/2
  In1/1 -> Compare Limit_Low_relop/1

== system gm_parallel_phase_voltages_per_switching_state_6_vnl/Phase_voltages_per_switching_state/Data Type Conversion1 ==
  In1 : Inport
  Data Type Conversion1 : DataTypeConversion  OutDataTypeStr=fixdt(1, 24, 11)  SampleTime=1e-08  SaturateOnIntegerOverflow=off  RndMeth=Floor
  Data Type Conversion1_pd1 : Delay  DelayLength=6
  Out1 : Outport
  wires:
  Data Type Conversion1_pd1/1 -> Out1/1
  Data Type Conversion1/1 -> Data Type Conversion1_pd1/1
  In1/1 -> Data Type Conversion1/1

== system gm_parallel_phase_voltages_per_switching_state_6_vnl/Phase_voltages_per_switching_state/Data Type Conversion6 ==
  In1 : Inport
  Data Type Conversion6 : DataTypeConversion  OutDataTypeStr=single  RndMeth=Nearest  SampleTime=1e-08  SaturateOnIntegerOverflow=off
  Data Type Conversion6_pd1 : Delay  DelayLength=6
  Out1 : Outport
  wires:
  Data Type Conversion6_pd1/1 -> Out1/1
  Data Type Conversion6/1 -> Data Type Conversion6_pd1/1
  In1/1 -> Data Type Conversion6/1

== system gm_parallel_phase_voltages_per_switching_state_6_vnl/Phase_voltages_per_switching_state/Detect Rise Positive ==
  note: U(k)
  note: Edge
  U : Inport  OutDataTypeStr=boolean  SampleTime=1e-08
  Delay Input1 : UnitDelay  Description=Store in Global RAM  DisableCoverage=on  InitialCondition=vinit  SampleTime=-1  HasFrameUpgradeWarning=on
  FixPt Relational Operator : RelationalOperator  Operator=>  OutDataTypeStr=boolean  ZeroCross=off  InputSameDT=off
  Positive : Subsystem  mask(Compare To Zero){relop=>, OutDataTypeStr=boolean, ZeroCross=off}
      mask prompts: relop "Simulink:masks:Operator_MP"; OutDataTypeStr "Simulink:masks:OutputDataType_MP"; ZeroCross "Simulink:masks:EnableZerocrossingDetection_MP"
      mask help: Simulink:masks:CompareToZero_MD
      mask init:
      | OutDataTypeStr = 'boolean';
      | ZeroCross = 'off';
      | blkName = 'parallel_phase_voltages_per_switching_state_6/Phase_voltages_per_switching_state/Detect Rise\nPositive/Positive';
      | relop = '>';
      | setValue = 'boolean';
      mask TypeOptions relop: == | ~= | < | <= | >= | >
      mask TypeOptions OutDataTypeStr: Simulink:masks:uint8 | Simulink:masks:boolean
      mask Callback ZeroCross: sl('zeroCrossEnable', gcbh);
      mask Display: disp([relop,' 0'])
  Y : Outport  SampleTime=1e-08
  wires:
  U/1 -> Positive/1(u)
  Positive/1(y) -> Delay Input1/1, FixPt Relational Operator/1
  FixPt Relational Operator/1 -> Y/1
  Delay Input1/1 -> FixPt Relational Operator/2

== system gm_parallel_phase_voltages_per_switching_state_6_vnl/Phase_voltages_per_switching_state/Detect Rise Positive1 ==
  note: U(k)
  note: Edge
  U : Inport  OutDataTypeStr=boolean  SampleTime=1e-08
  Delay Input1 : UnitDelay  Description=Store in Global RAM  DisableCoverage=on  InitialCondition=vinit  SampleTime=-1  HasFrameUpgradeWarning=on
  FixPt Relational Operator : RelationalOperator  Operator=>  OutDataTypeStr=boolean  ZeroCross=off  InputSameDT=off
  Positive : Subsystem  mask(Compare To Zero){relop=>, OutDataTypeStr=boolean, ZeroCross=off}
      mask prompts: relop "Simulink:masks:Operator_MP"; OutDataTypeStr "Simulink:masks:OutputDataType_MP"; ZeroCross "Simulink:masks:EnableZerocrossingDetection_MP"
      mask help: Simulink:masks:CompareToZero_MD
      mask init:
      | OutDataTypeStr = 'boolean';
      | ZeroCross = 'off';
      | blkName = 'parallel_phase_voltages_per_switching_state_6/Phase_voltages_per_switching_state/Detect Rise\nPositive1/Positive';
      | relop = '>';
      | setValue = 'boolean';
      mask TypeOptions relop: == | ~= | < | <= | >= | >
      mask TypeOptions OutDataTypeStr: Simulink:masks:uint8 | Simulink:masks:boolean
      mask Callback ZeroCross: sl('zeroCrossEnable', gcbh);
      mask Display: disp([relop,' 0'])
  Y : Outport  SampleTime=1e-08
  wires:
  U/1 -> Positive/1(u)
  Positive/1(y) -> Delay Input1/1, FixPt Relational Operator/1
  FixPt Relational Operator/1 -> Y/1
  Delay Input1/1 -> FixPt Relational Operator/2
